simulink library "rotorTorqueCtrl"  (R2022a)
settings: Solver=VariableStepAuto  StartTime=0.0  StopTime=10.0  RelTol=1e-3
undefined symbols (not defined in the file): rho, turbOpt, vhcl
libraries: matrix_library x1, sixDoFDynamicsCoupledFossenTurbDynamics x1, alphaBeta_ul x1, localApparentWind_ul x1
settings Model: Creator=adabney  LastModifiedBy=adabney

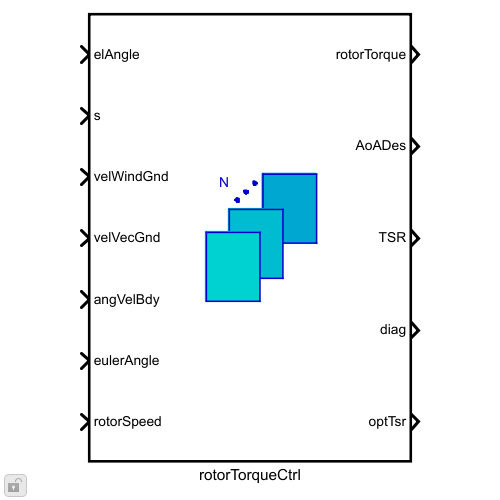
[thumbnail: Simulink's stored preview of the top-level diagram]
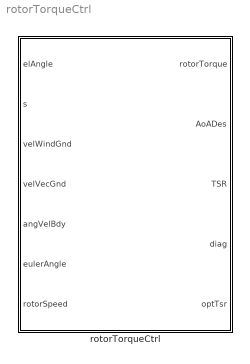
== system rotorTorqueCtrl ==
  rotorTorqueCtrl : Subsystem  TreatAsAtomicUnit=on  mask{turb_struct=vhcl.struct('OCT.turb'), rho=rho}
      mask prompts: turb_struct "Turbine Structures"; rho "Fluid Density"

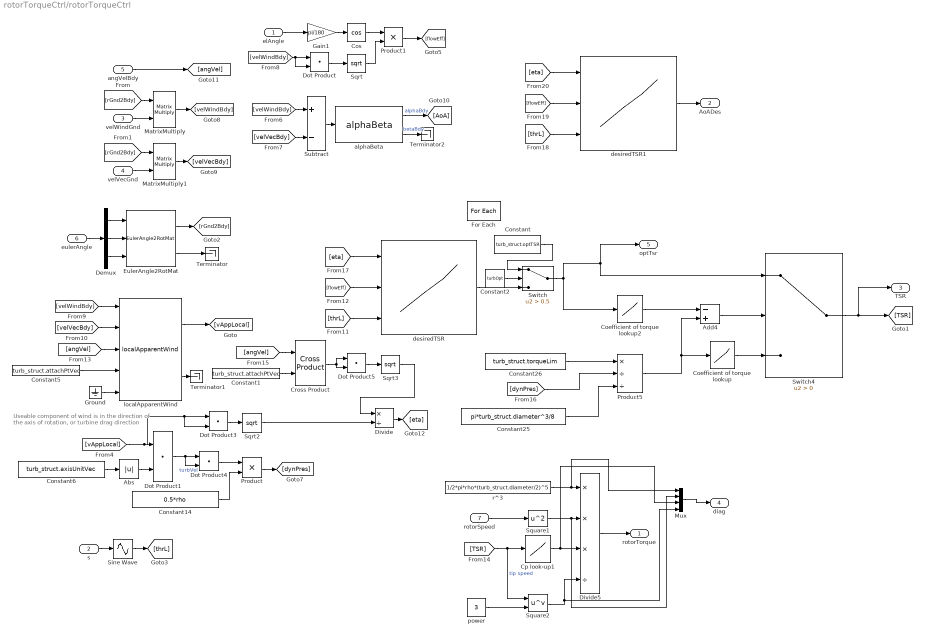
== system rotorTorqueCtrl/rotorTorqueCtrl ==
  note: Useable component of wind is in the direction of
      | the axis of rotation, or turbine drag direction
  elAngle : Inport
  s : Inport  Port=2
  velWindGnd : Inport  Port=3
  velVecGnd : Inport  Port=4
  angVelBdy : Inport  Port=5
  eulerAngle : Inport  Port=6
  rotorSpeed : Inport  Port=7  Partition=on  PartitionDimension=1  PartitionWidth=1  PartitionOffset=0
  Abs : Abs  SaturateOnIntegerOverflow=off
  Add4 : Sum  Inputs=-+
  Coefficient of torque lookup : Lookup_n-D  NumberOfTableDimensions=1  BreakpointsForDimension1=turb_struct.tauCoefLookup  Table=turb_struct.tauCoefTSR  InternalRulePriority=Speed  RndMeth=Simplest
  Coefficient of torque lookup2 : Lookup_n-D  NumberOfTableDimensions=1  BreakpointsForDimension1=turb_struct.tauCoefTSR(end:-1:1)  Table=turb_struct.tauCoefLookup(end:-1:1)  InternalRulePriority=Speed  RndMeth=Simplest
  Constant : Constant  Value=turb_struct.optTSR
  Constant1 : Constant  Value=turb_struct.attachPtVec
  Constant14 : Constant  Value=0.5*rho
  Constant2 : Constant  Value=turbOpt
  Constant25 : Constant  Value=pi*turb_struct.diameter^3/8
  Constant26 : Constant  Value=turb_struct.torqueLim
  Constant5 : Constant  Value=turb_struct.attachPtVec
  Constant6 : Constant  Value=turb_struct.axisUnitVec
  Cos : Trigonometry  Operator=cos
  Cp look-up1 : Lookup_n-D  NumberOfTableDimensions=1  BreakpointsForDimension1=turb_struct.RPMref  Table=turb_struct.CpLookup  InternalRulePriority=Speed  RndMeth=Simplest
  Cross Product : matrix_library/Cross Product
      settings: SourceProductBaseCode=SL
  Demux : Demux  Outputs=3
  Divide : Product  Inputs=*/
  Divide5 : Product  Inputs=***/
  Dot Product{,1,3..5} (5 alike) : DotProduct  OutDataTypeStr=Inherit: Inherit via internal rule
  EulerAngle2RotMat : sixDoFDynamicsCoupledFossenTurbDynamics/sixDoFDynamicsCoupledFossenTurbDynamics/EulerAngle2RotMat  SystemSampleTime=-1  VariantActivationTime=update diagram  Latency=0  AutoFrameSizeCalculation=off
  For Each : ForEach  DisableCoverage=on  IterateSubsysMaskParameter=on,off  SubsysMaskParameterIterationDimension=2,1  SubsysMaskParameterIterationStepSize=1,1
  Gain1 : Gain  Gain=pi/180
  Ground : Ground
  MatrixMultiply : Product  Multiplication=Matrix(*)
  MatrixMultiply1 : Product  Multiplication=Matrix(*)
  Mux : Mux
  Product : Product
  Product1 : Product
  Product5 : Product  Inputs=*//
  Sine Wave : Sin  TimeSource=Use external signal  Amplitude=10  Bias=80  Frequency=4*pi  Phase=pi/2  SampleTime=0
  Sqrt : Sqrt
  Sqrt2 : Sqrt
  Sqrt3 : Sqrt
  Square1 : Math  Operator=square
  Square2 : Math  Operator=pow
  Subtract : Sum  Inputs=+-
  Switch : Switch  Criteria=u2 > Threshold  Threshold=0.5  SaturateOnIntegerOverflow=off  InputSameDT=off
  Switch4 : Switch  Criteria=u2 > Threshold  SaturateOnIntegerOverflow=off  InputSameDT=off
  Terminator : Terminator
  Terminator1 : Terminator
  Terminator2 : Terminator
  alphaBeta : alphaBeta_ul/alphaBeta  SystemSampleTime=-1  VariantActivationTime=update diagram  Latency=0  AutoFrameSizeCalculation=off
  desiredTSR : Lookup_n-D  NumberOfTableDimensions=3  BreakpointsForDimension1=turb_struct.etaLookup  BreakpointsForDimension2=turb_struct.velWLookup  BreakpointsForDimension3=turb_struct.thrLookup  Table=turb_struct.tsrLookup  InternalRulePriority=Speed  RndMeth=Simplest
      settings: InputPortMap=u0,u1,u2
  desiredTSR1 : Lookup_n-D  NumberOfTableDimensions=3  BreakpointsForDimension1=turb_struct.etaLookup  BreakpointsForDimension2=turb_struct.velWLookup  BreakpointsForDimension3=turb_struct.thrLookup  Table=turb_struct.AoALookup  InternalRulePriority=Speed  RndMeth=Simplest
      settings: InputPortMap=u0,u1,u2
  localApparentWind : localApparentWind_ul/localApparentWind  SystemSampleTime=-1  VariantActivationTime=update diagram  Latency=0  AutoFrameSizeCalculation=off
  power : Constant  Value=3
  r^3 : Constant  Value=1/2*pi*rho*(turb_struct.diameter/2)^5
  rotorTorque : Outport  ConcatenationDimension=1
  AoADes : Outport  Port=2  ConcatenationDimension=1
  TSR : Outport  Port=3  ConcatenationDimension=1
  diag : Outport  Port=4  ConcatenationDimension=1
  optTsr : Outport  Port=5  ConcatenationDimension=1
  wires:
  Constant25/1 -> Product5/3
  desiredTSR/1 -> Switch/3
  Coefficient of torque lookup2/1 -> Add4/1
  [dynPres] -> Product5/2
  Product5/1 -> Add4/2, Coefficient of torque lookup/1
  Switch4/1 -> TSR/1, [TSR]
  Constant26/1 -> Product5/1
  Add4/1 -> Switch4/2
  Coefficient of torque lookup/1 -> Switch4/3
  [vAppLocal] -> Dot Product3/2, Dot Product3/1, Dot Product1/1
  Constant6/1 -> Abs/1
  Abs/1 -> Dot Product1/2
  Dot Product4/1 -> Product/1
  Product/1 -> [dynPres]
  Dot Product1/1 -> Dot Product4/1, Dot Product4/2  "turbVel"
  Ground/1 -> localApparentWind/5
  Constant5/1 -> localApparentWind/4
  Constant14/1 -> Product/2
  localApparentWind/1 -> [vAppLocal]
  localApparentWind/2 -> Terminator1/1
  [angVel] -> localApparentWind/3
  EulerAngle2RotMat/1 -> [rGnd2Bdy]
  Demux/3 -> EulerAngle2RotMat/3
  Demux/1 -> EulerAngle2RotMat/1
  EulerAngle2RotMat/2 -> Terminator/1
  eulerAngle/1 -> Demux/1
  Demux/2 -> EulerAngle2RotMat/2
  [velWindBdy] -> localApparentWind/1
  [velVecBdy] -> localApparentWind/2
  power/1 -> Square2/2
  Cp look-up1/1 -> Mux/3, Divide5/3
  Square1/1 -> Mux/2, Divide5/2
  Square2/1 -> Mux/4, Divide5/4
  Divide5/1 -> rotorTorque/1
  r^3/1 -> Mux/1, Divide5/1
  [TSR] -> Square2/1, Cp look-up1/1  "tip speed"
  rotorSpeed/1 -> Square1/1
  Sine Wave/1 -> [thrL]
  [rGnd2Bdy] -> MatrixMultiply1/1
  [rGnd2Bdy] -> MatrixMultiply/1
  velVecGnd/1 -> MatrixMultiply1/2
  velWindGnd/1 -> MatrixMultiply/2
  MatrixMultiply/1 -> [velWindBdy]
  MatrixMultiply1/1 -> [velVecBdy]
  [velVecBdy] -> Subtract/2
  [velWindBdy] -> Subtract/1
  Subtract/1 -> alphaBeta/1
  alphaBeta/2 -> Terminator2/1  "betaBdy"
  alphaBeta/1 -> [AoA]  "alphaBdy"
  Product1/1 -> [flowEff]
  Sqrt/1 -> Product1/2
  Gain1/1 -> Cos/1
  Cos/1 -> Product1/1
  Dot Product/1 -> Sqrt/1
  elAngle/1 -> Gain1/1
  [velWindBdy] -> Dot Product/2, Dot Product/1
  s/1 -> Sine Wave/1
  [thrL] -> desiredTSR/3
  [flowEff] -> desiredTSR/2
  Dot Product3/1 -> Sqrt2/1
  angVelBdy/1 -> [angVel]
  [angVel] -> Cross Product/1
  Constant1/1 -> Cross Product/2
  Cross Product/1 -> Dot Product5/1, Dot Product5/2
  Sqrt2/1 -> Divide/2
  Sqrt3/1 -> Divide/1
  Dot Product5/1 -> Sqrt3/1
  Divide/1 -> [eta]
  [eta] -> desiredTSR/1
  [eta] -> desiredTSR1/1
  [flowEff] -> desiredTSR1/2
  [thrL] -> desiredTSR1/3
  desiredTSR1/1 -> AoADes/1
  Mux/1 -> diag/1
  Switch/1 -> Switch4/1, optTsr/1, Coefficient of torque lookup2/1
  Constant/1 -> Switch/1
  Constant2/1 -> Switch/2
